simulink model "SteeringColumn"  (R2023a)
settings: Solver=VariableStepAuto  StartTime=0.0  StopTime=10.0  RelTol=1e-3
undefined symbols (not defined in the file): B_total, c, J_total, T_f_total
settings Model: Creator=Tan_Tram  LastModifiedBy=Tan_Tram

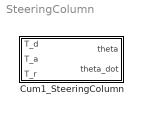
== system SteeringColumn ==
  Cum1_SteeringColumn : Subsystem

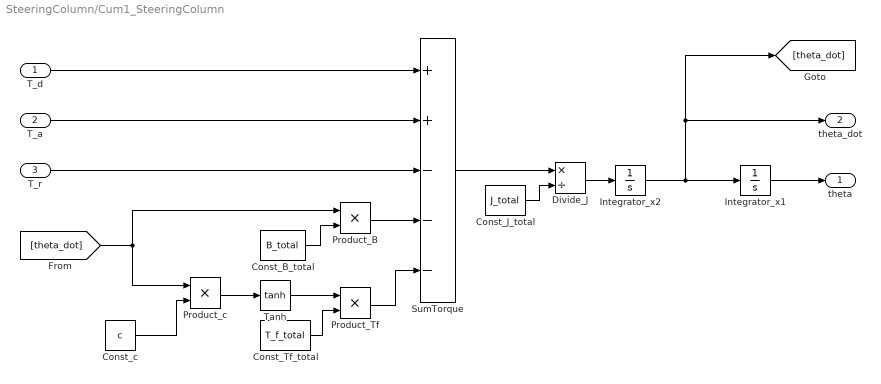
== system SteeringColumn/Cum1_SteeringColumn ==
  T_d : Inport
  T_a : Inport  Port=2
  T_r : Inport  Port=3
  Const_B_total : Constant  Value=B_total
  Const_J_total : Constant  Value=J_total
  Const_Tf_total : Constant  Value=T_f_total
  Const_c : Constant  Value=c
  Divide_J : Product  Inputs=*/
  Integrator_x1 : Integrator
  Integrator_x2 : Integrator
  Product_B : Product
  Product_Tf : Product
  Product_c : Product
  SumTorque : Sum  Inputs=++---
  Tanh : Trigonometry  Operator=tanh
  theta : Outport
  theta_dot : Outport  Port=2
  wires:
  T_d/1 -> SumTorque/1
  T_a/1 -> SumTorque/2
  T_r/1 -> SumTorque/3
  Integrator_x2/1 -> Integrator_x1/1, [theta_dot], theta_dot/1
  Const_B_total/1 -> Product_B/2
  Product_B/1 -> SumTorque/4
  Const_c/1 -> Product_c/2
  Product_c/1 -> Tanh/1
  Tanh/1 -> Product_Tf/1
  Const_Tf_total/1 -> Product_Tf/2
  Product_Tf/1 -> SumTorque/5
  SumTorque/1 -> Divide_J/1
  Const_J_total/1 -> Divide_J/2
  Divide_J/1 -> Integrator_x2/1
  Integrator_x1/1 -> theta/1
  [theta_dot] -> Product_c/1, Product_B/1
